simulink model "BLDC_motor"  (R2020b)
settings: Solver=VariableStepAuto  StartTime=0.0  StopTime=10.0  RelTol=1e-3
undefined symbols (not defined in the file): Fw, J, L, lambda, R
libraries: simulink x2
settings Model: Creator=Shubham  LastModifiedBy=Shubham

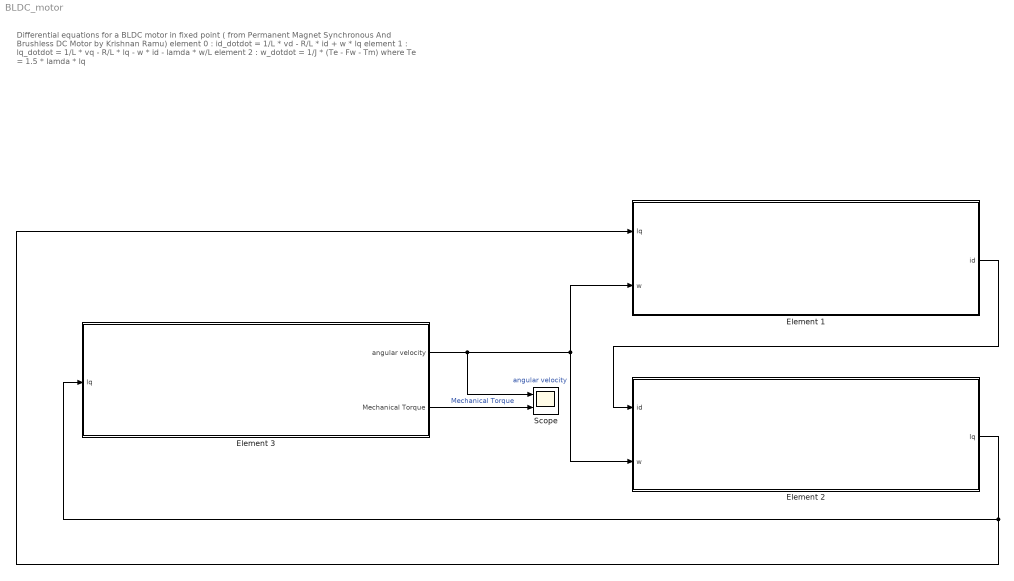
== system BLDC_motor ==
  note: Differential equations for a BLDC motor in fixed point
      | ( from Permanent Magnet Synchronous And Brushless DC Motor by Krishnan Ramu)
      |
      | element 0 : id_dotdot = 1/L * vd - R/L * id + w * lq
      |
      | element 1 : lq_dotdot = 1/L * vq - R/L * lq - w * id - lamda * w/L
      |
      | element 2 : w_dotdot = 1/J * (Te - Fw - Tm) where Te = 1.5 * lamda * lq
  Element 1 : Subsystem
  Element 2 : Subsystem
  Element 3 : Subsystem
  Scope : Scope  NumInputPorts=2
  wires:
  Element 3/1(angular velocity) -> Scope/1, Element 1/2(w), Element 2/2(w)  "angular velocity"
  Element 1/1(id) -> Element 2/1(id)
  Element 2/1(lq) -> Element 1/1(lq), Element 3/1(lq)
  Element 3/2(Mechanical Torque) -> Scope/2  "Mechanical Torque"

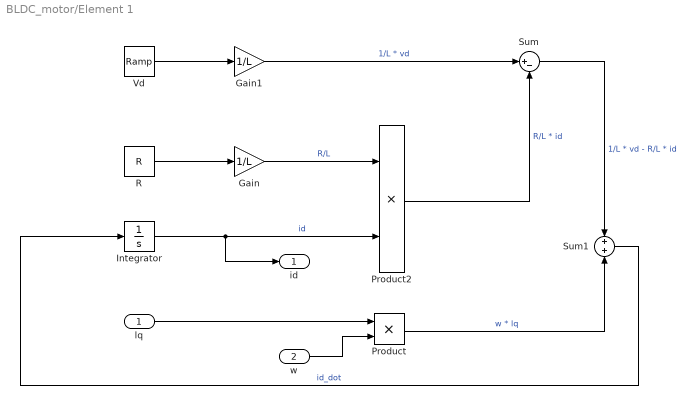
== system BLDC_motor/Element 1 ==
  lq : Inport
  w : Inport  Port=2
  Gain : Gain  Gain=1/L
  Gain1 : Gain  Gain=1/L
  Integrator : Integrator
  Product : Product
  Product2 : Product
  R : Constant  Value=R
  Sum : Sum  Inputs=|+-
  Sum1 : Sum
  Vd : simulink/Sources/Ramp  slope=1  start=0  InitialOutput=0
  id : Outport
  wires:
  Sum/1 -> Sum1/1  "1/L * vd - R/L * id"
  Sum1/1 -> Integrator/1  "id_dot"
  Gain/1 -> Product2/1  "R/L"
  R/1 -> Gain/1
  Integrator/1 -> id/1, Product2/2  "id"
  Product2/1 -> Sum/2  "R/L * id"
  Product/1 -> Sum1/2  "w * lq"
  Gain1/1 -> Sum/1  "1/L * vd"
  lq/1 -> Product/1
  w/1 -> Product/2
  Vd/1 -> Gain1/1

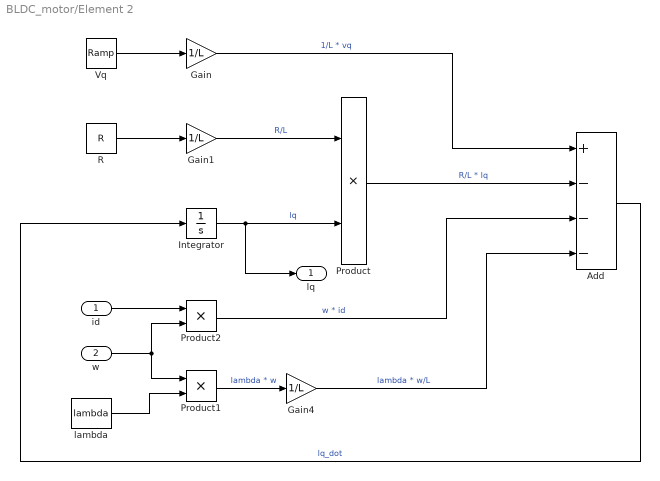
== system BLDC_motor/Element 2 ==
  id : Inport
  w : Inport  Port=2
  Add : Sum  Inputs=+---
  Gain : Gain  Gain=1/L
  Gain1 : Gain  Gain=1/L
  Gain4 : Gain  Gain=1/L
  Integrator : Integrator
  Product : Product
  Product1 : Product
  Product2 : Product
  R : Constant  Value=R
  Vq : simulink/Sources/Ramp  slope=1  start=0  InitialOutput=0
  lambda : Constant  Value=lambda
  lq : Outport
  wires:
  Integrator/1 -> lq/1, Product/2  "lq"
  Product2/1 -> Add/3  "w * id"
  Gain/1 -> Add/1  "1/L * vq"
  Product/1 -> Add/2  "R/L * lq"
  Add/1 -> Integrator/1  "lq_dot"
  Gain4/1 -> Add/4  "lambda * w/L"
  R/1 -> Gain1/1
  Product1/1 -> Gain4/1  "lambda * w"
  lambda/1 -> Product1/2
  Gain1/1 -> Product/1  "R/L"
  id/1 -> Product2/1
  w/1 -> Product2/2, Product1/1
  Vq/1 -> Gain/1

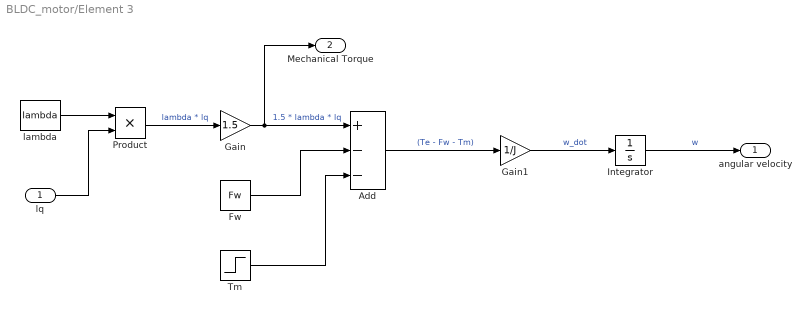
== system BLDC_motor/Element 3 ==
  lq : Inport
  Add : Sum  Inputs=+--
  Fw : Constant  Value=Fw
  Gain : Gain  Gain=1.5
  Gain1 : Gain  Gain=1/J
  Integrator : Integrator
  Product : Product
  Tm : Step  SampleTime=0
  lambda : Constant  Value=lambda
  angular velocity : Outport
  Mechanical Torque : Outport  Port=2
  wires:
  Gain1/1 -> Integrator/1  "w_dot"
  Gain/1 -> Mechanical Torque/1, Add/1  "1.5 * lambda * lq"
  Tm/1 -> Add/3
  Add/1 -> Gain1/1  "(Te - Fw - Tm)"
  Integrator/1 -> angular velocity/1  "w"
  lambda/1 -> Product/1
  lq/1 -> Product/2
  Product/1 -> Gain/1  "lambda * lq"
  Fw/1 -> Add/2
